simulink model "zad6"  (R2023a)
settings: Solver=VariableStepAuto  StartTime=0.0  StopTime=100.0  RelTol=1e-3
model workspace (MAT data in the model file):
  T1 = Simulink.Parameter
  T1.Value = 8
  T1.DataType = 'auto'
  T1.Complexity = 'real'
  T1.Dimensions = [1 1]
  T2 = Simulink.Parameter
  T2.Value = 9
  T2.DataType = 'auto'
  T2.Complexity = 'real'
  T2.Dimensions = [1 1]
values from neighbouring files (symbols this model uses):
  K = 1    [zad10.m]    (also in zad2.m; zad3.m)
  T1 = 9    [zad10.m]
  T2 = 8    [zad10.m]
undefined symbols (not defined in the file or in its folder): DiscIntNeverNeededParam
settings Model: Creator=pkutyl  LastModifiedBy=pkutyl

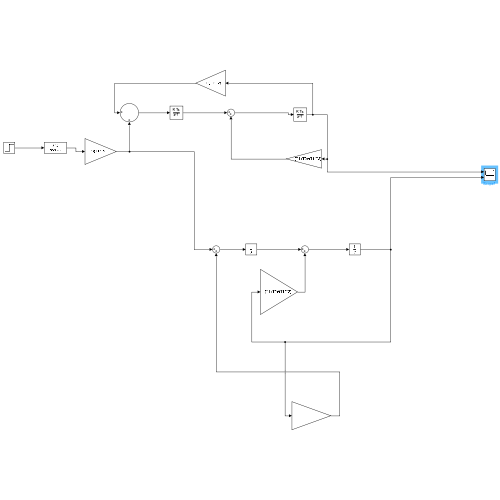
[thumbnail: Simulink's stored preview of the top-level diagram]
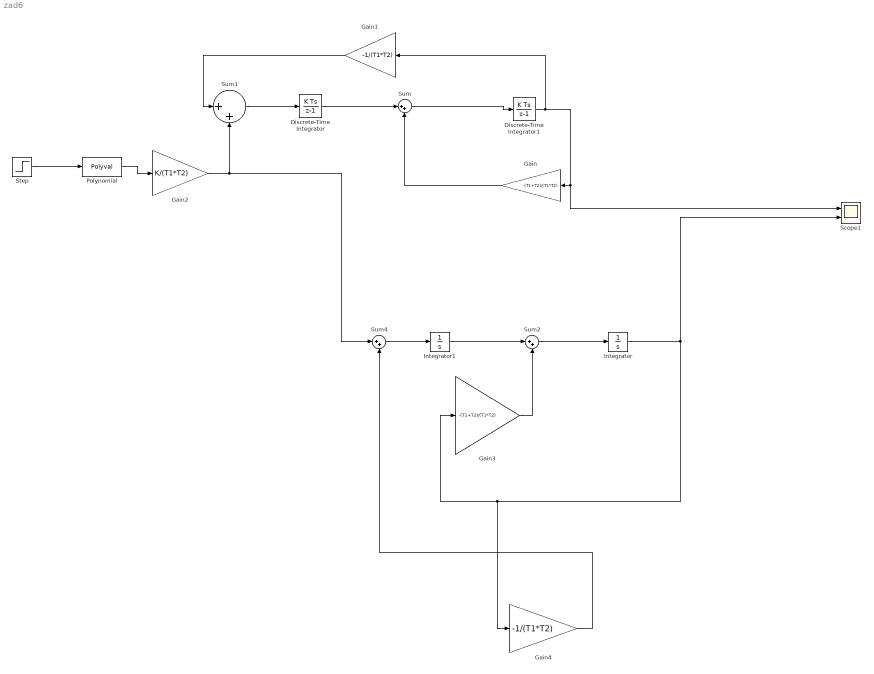
== system zad6 ==
  Discrete-Time Integrator : DiscreteIntegrator  SampleTime=3  ICPrevOutput=DiscIntNeverNeededParam  ICPrevScaledInput=DiscIntNeverNeededParam
  Discrete-Time Integrator1 : DiscreteIntegrator  SampleTime=3  ICPrevOutput=DiscIntNeverNeededParam  ICPrevScaledInput=DiscIntNeverNeededParam
  Gain : Gain  Gain=-(T1+T2)/(T1*T2)
  Gain1 : Gain  Gain=-1/(T1*T2)
  Gain2 : Gain  Gain=K/(T1*T2)
  Gain3 : Gain  Gain=-(T1+T2)/(T1*T2)
  Gain4 : Gain  Gain=-1/(T1*T2)
  Integrator : Integrator
  Integrator1 : Integrator
  Polynomial : Polyval  Coefs=[-0.41,-0.41,-0.86,-0.8]
  Scope1 : Scope  NumInputPorts=2
  Step : Step  SampleTime=1
  Sum{,1..2,4} (4 alike) : Sum  Inputs=|++
  wires:
  Sum/1 -> Discrete-Time Integrator1/1
  Gain1/1 -> Sum1/1
  Gain/1 -> Sum/2
  Sum1/1 -> Discrete-Time Integrator/1
  Polynomial/1 -> Gain2/1
  Step/1 -> Polynomial/1
  Discrete-Time Integrator1/1 -> Gain1/1, Scope1/1, Gain/1
  Discrete-Time Integrator/1 -> Sum/1
  Integrator/1 -> Scope1/2, Gain4/1, Gain3/1
  Integrator1/1 -> Sum2/1
  Gain3/1 -> Sum2/2
  Sum4/1 -> Integrator1/1
  Sum2/1 -> Integrator/1
  Gain4/1 -> Sum4/2
  Gain2/1 -> Sum4/1, Sum1/2
